simulink model "Joystick_Input"  (R2024b)
settings: Solver=VariableStepAuto  StartTime=0.0  StopTime=10.0  RelTol=1e-3
libraries: aerolibconvert2 x1, aerolibanimutils x1
settings Model: Creator=annaf  LastModifiedBy=annaf

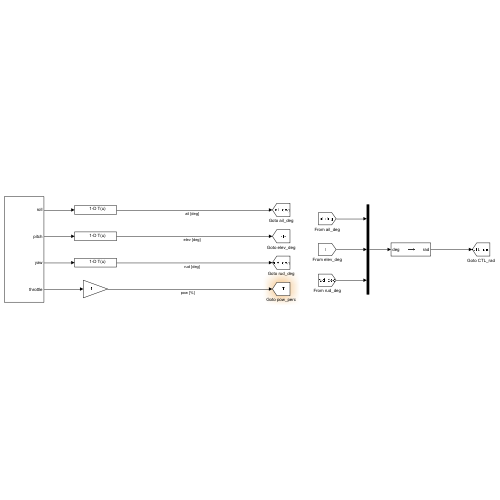
[thumbnail: Simulink's stored preview of the top-level diagram]
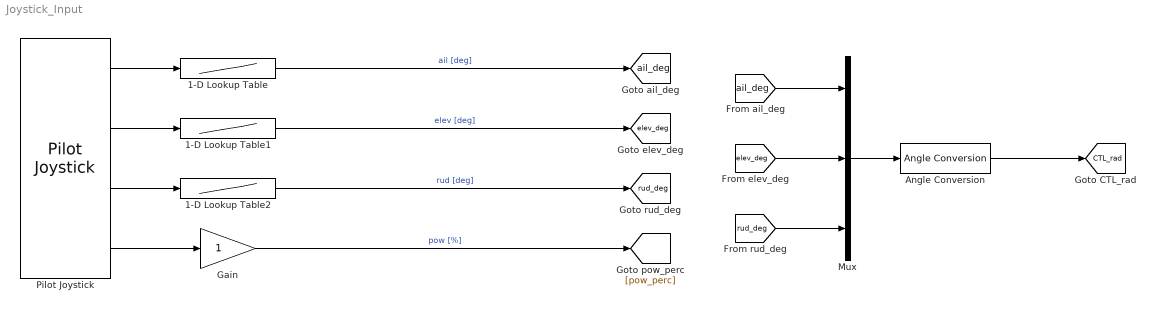
== system Joystick_Input ==
  1-D Lookup Table : Lookup_n-D  NumberOfTableDimensions=1  BreakpointsForDimension1=[-5:5]  Table=tanh([-5:5])  InternalRulePriority=Speed  RndMeth=Simplest
  1-D Lookup Table1 : Lookup_n-D  NumberOfTableDimensions=1  BreakpointsForDimension1=[-5:5]  Table=tanh([-5:5])  InternalRulePriority=Speed  RndMeth=Simplest
  1-D Lookup Table2 : Lookup_n-D  NumberOfTableDimensions=1  BreakpointsForDimension1=[-5:5]  Table=tanh([-5:5])  InternalRulePriority=Speed  RndMeth=Simplest
  Angle Conversion : aerolibconvert2/Angle Conversion  IU=deg  OU=rad
  Gain : Gain
  Mux : Mux  Inputs=3
  Pilot Joystick : aerolibanimutils/Pilot Joystick  JoystickID=Joystick1  OutputConfiguration=FourAxis  SampleTime=1/30
  tag scope: CTL_rad=global, ail_deg=global, elev_deg=global, rud_deg=global
  wires:
  Pilot Joystick/1 -> 1-D Lookup Table/1
  Pilot Joystick/2 -> 1-D Lookup Table1/1
  Pilot Joystick/3 -> 1-D Lookup Table2/1
  Pilot Joystick/4 -> Gain/1
  1-D Lookup Table/1 -> [ail_deg]  "ail [deg]"
  1-D Lookup Table1/1 -> [elev_deg]  "elev [deg]"
  1-D Lookup Table2/1 -> [rud_deg]  "rud [deg]"
  Gain/1 -> [pow_perc]  "pow [%]"
  [ail_deg] -> Mux/1
  [elev_deg] -> Mux/2
  [rud_deg] -> Mux/3
  Mux/1 -> Angle Conversion/1
  Angle Conversion/1 -> [CTL_rad]
